simulink model "HDLRxPayload"  (R2024a)
settings: Solver=FixedStepDiscrete  StartTime=0.0  StopTime=stopTime  RelTol=1e-3
values from neighbouring files (symbols this model uses):
  payloadRxLLR = ofdmDemodulate(payloadTx, payloadBitsPerSubcarrier, payloadCyclicPrefixLen, nullIdx, payloadScramblerInit, true)    [testRxPayload.m]
  validIn = true(size(payloadRxLLR))    [testRxPayload.m]
undefined symbols (not defined in the file or in its folder): CONST, totalPayloadFecBlocks
libraries: hdlsllib x9, dspsrcs4 x8, HDL_ieee_8021513 x2, whdlutilities x1
settings Model: DataTypeOverride=Off  SimulationMode=accelerator  Creator=cotti  LastModifiedBy=cotti
settings OptimizationCC: BlockReduction=off  ConditionallyExecuteInputs=off  DefaultParameterBehavior=Inlined  InheritOutputTypeSmallerThanSingle=on
settings DebuggingCC: AlgebraicLoopMsg=error  ArtificialAlgebraicLoopMsg=error  SingleTaskRateTransMsg=error  UnconnectedInputMsg=warning  UnconnectedOutputMsg=warning  UnconnectedLineMsg=warning
settings HardwareCC: ProdBitPerPointer=32  ProdBitPerSizeT=32  ProdBitPerPtrDiffT=32  ProdLargestAtomicFloat=None  ProdIntDivRoundTo=Undefined  ProdEndianess=Unspecified  ProdWordSize=32  ProdHWDeviceType=ASIC/FPGA->ASIC/FPGA  TargetBitPerLong=64  TargetBitPerPointer=64  TargetBitPerSizeT=64  TargetBitPerPtrDiffT=64  TargetLongLongMode=on  TargetIntDivRoundTo=Zero  TargetEndianess=LittleEndian  TargetWordSize=64  TargetHWDeviceType=Custom Processor->MATLAB Host Computer  ProdEqTarget=off

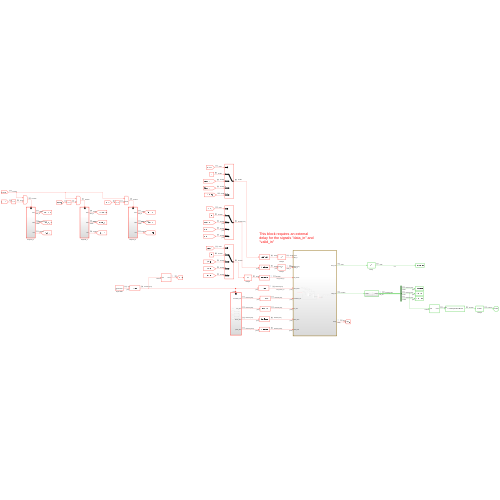
[thumbnail: Simulink's stored preview of the top-level diagram]
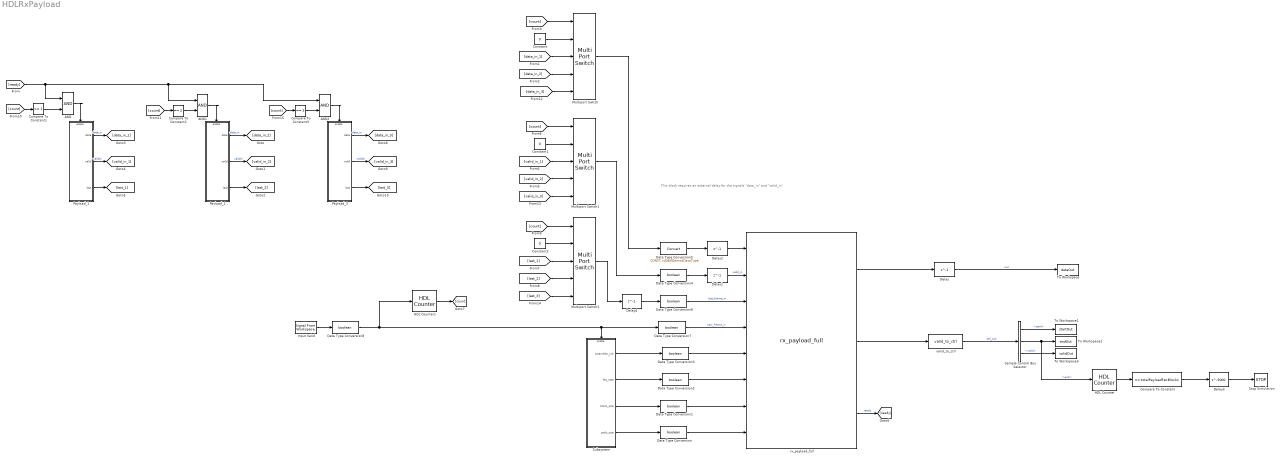
== system HDLRxPayload ==
  note: This block requires an external delay for the signals "data_in" and "valid_in"
  AND : Logic  IconShape=distinctive  AllPortsSameDT=off  OutDataTypeStr=boolean
  AND1 : Logic  IconShape=distinctive  AllPortsSameDT=off  OutDataTypeStr=boolean
  AND2 : Logic  IconShape=distinctive  AllPortsSameDT=off  OutDataTypeStr=boolean
  Compare To Constant : hdlsllib/Logic and Bit Operations/Compare To Constant  relop===  const=totalPayloadFecBlocks  OutDataTypeStr=boolean
  Compare To Constant1 : hdlsllib/Logic and Bit Operations/Compare To Constant  relop===  const=1  OutDataTypeStr=boolean
  Compare To Constant2 : hdlsllib/Logic and Bit Operations/Compare To Constant  relop===  const=2  OutDataTypeStr=boolean
  Compare To Constant3 : hdlsllib/Logic and Bit Operations/Compare To Constant  relop===  const=3  OutDataTypeStr=boolean
  Constant : Constant  Value=0  OutDataTypeStr=Inherit: Inherit via back propagation  SampleTime=-1
  Constant1 : Constant  Value=0  OutDataTypeStr=Inherit: Inherit via back propagation  SampleTime=-1
  Constant2 : Constant  Value=0  OutDataTypeStr=Inherit: Inherit via back propagation  SampleTime=-1
  Data Type Conversion{,1..4,6..8} (8 alike) : DataTypeConversion  OutDataTypeStr=boolean  SaturateOnIntegerOverflow=off  RndMeth=Floor
  Data Type Conversion5 : DataTypeConversion  OutDataTypeStr=CONST.rxQAMDemodDataType  SaturateOnIntegerOverflow=off  RndMeth=Floor
  Delay{,1..2,4} (4 alike) : Delay  DelayLength=1  InitialCondition=0  UseCircularBuffer=on
  Delay3 : Delay  DelayLength=5000  InitialCondition=0  UseCircularBuffer=on
  HDL Counter : hdlsllib/Sources/HDL Counter  CountType=Free running  CountInit=0  CountStep=1  CountMax=25  CountFromType=Initial value  CountFrom=0  CountResetPort=off  CountLoadPort=off  CountEnbPort=on  CountDirPort=off  CountHitOutputPort=off  CountDataType=Unsigned  CountWordLen=32  CountFracLen=0  CountSampTime=1
  HDL Counter1 : hdlsllib/Sources/HDL Counter  CountType=Free running  CountInit=0  CountStep=1  CountMax=25  CountFromType=Initial value  CountFrom=0  CountResetPort=off  CountLoadPort=off  CountEnbPort=on  CountDirPort=off  CountHitOutputPort=off  CountDataType=Unsigned  CountWordLen=8  CountFracLen=0  CountSampTime=1
  Input Valid : dspsrcs4/Signal From Workspace  X=newFrame  Ts=1/(2*CONST.fPHY)  nsamps=1  OutputAfterFinalValue=Setting to zero  ignoreOrWarnInputAndFrameLengths=off  OutputFrames=off
  Multiport Switch : MultiPortSwitch  DataPortOrder=Zero-based contiguous  Inputs=4  zeroidx=on  SaturateOnIntegerOverflow=off  InputSameDT=off
  Multiport Switch1 : MultiPortSwitch  DataPortOrder=Zero-based contiguous  Inputs=4  zeroidx=on  SaturateOnIntegerOverflow=off  InputSameDT=off
  Multiport Switch2 : MultiPortSwitch  DataPortOrder=Zero-based contiguous  Inputs=4  zeroidx=on  SaturateOnIntegerOverflow=off  InputSameDT=off
  Payload_1 : Subsystem  TreatAsAtomicUnit=on
  Payload_2 : Subsystem  TreatAsAtomicUnit=on
  Payload_3 : Subsystem  TreatAsAtomicUnit=on
  Sample Control Bus Selector : whdlutilities/Sample Control Bus Selector  OutputSignals=start,end,valid
  Stop Simulation : Stop
  Subsystem : Subsystem
  To Workspace : ToWorkspace  VariableName=dataOut  SampleTime=4/CONST.fPHY
      settings: Save2DSignal=2-D array (concatenate along first dimension)
  To Workspace1 : ToWorkspace  VariableName=startOut  SampleTime=4/CONST.fPHY
      settings: Save2DSignal=2-D array (concatenate along first dimension)
  To Workspace2 : ToWorkspace  VariableName=endOut  SampleTime=4/CONST.fPHY
      settings: Save2DSignal=2-D array (concatenate along first dimension)
  To Workspace3 : ToWorkspace  VariableName=validOut  SampleTime=4/CONST.fPHY
      settings: Save2DSignal=2-D array (concatenate along first dimension)
  rx_payload_full : HDL_ieee_8021513/rx_payload_full  SystemSampleTime=-1  VariantActivationTime=update diagram  AllowFlexibleInterface=on  Latency=0  AutoFrameSizeCalculation=off
      settings: SourceProductName=HDL IEEE 8021513
  valid_to_ctrl : HDL_ieee_8021513/valid_to_ctrl  SystemSampleTime=-1  VariantActivationTime=update diagram  AllowFlexibleInterface=on  Latency=0  AutoFrameSizeCalculation=off
      settings: SourceProductName=HDL IEEE 8021513
  wires:
  Sample Control Bus Selector/2 -> HDL Counter/1, To Workspace2/1  "<end>"
  Delay/1 -> To Workspace/1  "out"
  Sample Control Bus Selector/1 -> To Workspace1/1  "<start>"
  Sample Control Bus Selector/3 -> To Workspace3/1  "<valid>"
  valid_to_ctrl/1 -> Sample Control Bus Selector/1  "ctrl_out"
  rx_payload_full/2 -> valid_to_ctrl/1
  rx_payload_full/1 -> Delay/1
  Data Type Conversion/1 -> rx_payload_full/8
  Data Type Conversion1/1 -> rx_payload_full/7
  Data Type Conversion2/1 -> rx_payload_full/6
  Data Type Conversion3/1 -> rx_payload_full/5
  Data Type Conversion4/1 -> Delay1/1
  Data Type Conversion5/1 -> Delay2/1
  Data Type Conversion6/1 -> rx_payload_full/3  "last_frame_in"
  Data Type Conversion7/1 -> rx_payload_full/4  "new_frame_in"
  Delay2/1 -> rx_payload_full/1
  Delay1/1 -> rx_payload_full/2  "valid_in"
  HDL Counter/1 -> Compare To Constant/1
  Compare To Constant/1 -> Delay3/1
  Subsystem/1(scrambler_init) -> Data Type Conversion3/1
  Subsystem/2(fec_rate) -> Data Type Conversion2/1
  Subsystem/3(block_size) -> Data Type Conversion1/1
  Subsystem/4(psdu_size) -> Data Type Conversion/1
  Input Valid/1 -> Data Type Conversion8/1
  Delay3/1 -> Stop Simulation/1
  Payload_2/1(data) -> [data_in_2]  "data_in"
  Payload_2/2(valid) -> [valid_in_2]  "validIn"
  Payload_2/3(last) -> [last_2]
  Payload_1/1(data) -> [data_in_1]  "data_in"
  Payload_1/2(valid) -> [valid_in_1]  "validIn"
  Payload_1/3(last) -> [last_1]
  rx_payload_full/3 -> [ready]  "ready"
  [data_in_1] -> Multiport Switch/3
  [data_in_2] -> Multiport Switch/4
  Constant/1 -> Multiport Switch/2
  Multiport Switch/1 -> Data Type Conversion5/1
  HDL Counter1/1 -> [count]
  [count] -> Multiport Switch/1
  Constant1/1 -> Multiport Switch1/2
  [valid_in_2] -> Multiport Switch1/4
  [valid_in_1] -> Multiport Switch1/3
  [count] -> Multiport Switch1/1
  Constant2/1 -> Multiport Switch2/2
  [last_2] -> Multiport Switch2/4
  [last_1] -> Multiport Switch2/3
  [count] -> Multiport Switch2/1
  Multiport Switch2/1 -> Delay4/1
  Multiport Switch1/1 -> Data Type Conversion4/1
  AND/1 -> Payload_1/Enable
  AND1/1 -> Payload_2/Enable
  Compare To Constant1/1 -> AND/2
  Compare To Constant2/1 -> AND1/2
  [count] -> Compare To Constant1/1
  [count] -> Compare To Constant2/1
  Data Type Conversion8/1 -> HDL Counter1/1, Subsystem/Enable, Data Type Conversion7/1
  [data_in_3] -> Multiport Switch/5
  [valid_in_3] -> Multiport Switch1/5
  [last_3] -> Multiport Switch2/5
  Payload_3/3(last) -> [last_3]
  Payload_3/1(data) -> [data_in_3]  "data_in"
  Payload_3/2(valid) -> [valid_in_3]  "validIn"
  Compare To Constant3/1 -> AND2/2
  [count] -> Compare To Constant3/1
  [ready] -> AND/1, AND2/1, AND1/1
  AND2/1 -> Payload_3/Enable
  Delay4/1 -> Data Type Conversion6/1

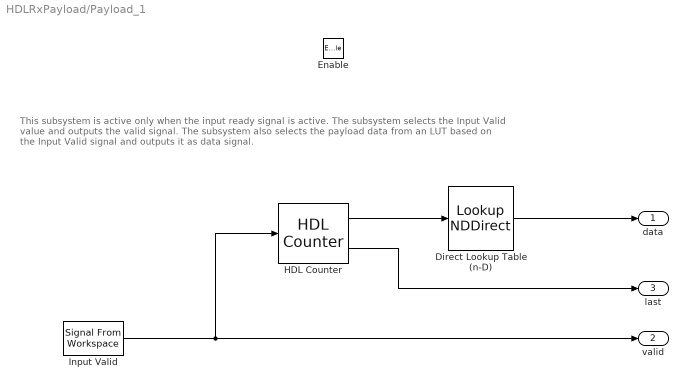
== system HDLRxPayload/Payload_1 ==
  note: This subsystem is active only when the input ready signal is active. The subsystem selects the Input Valid value and outputs the valid signal.
      | The subsystem also selects the payload data from an LUT based on the Input Valid signal and outputs it as data signal.
  Enable : EnablePort
  Direct Lookup Table (n-D) : LookupNDDirect  NumberOfTableDimensions=1  Table=payloadRxLLR{1}  DiagnosticForOutOfRangeInput=Error  TableDataTypeStr=double
  HDL Counter : hdlsllib/Sources/HDL Counter  CountType=Count limited  CountInit=0  CountStep=1  CountMax=length(payloadRxLLR{1}) -1  CountFromType=Initial value  CountFrom=0  CountResetPort=off  CountLoadPort=off  CountEnbPort=on  CountDirPort=off  CountHitOutputPort=on  CountDataType=Unsigned  CountWordLen=nextpow2(length(payloadRxLLR{1}))  CountFracLen=0  CountSampTime=1
  Input Valid : dspsrcs4/Signal From Workspace  X=validIn{1}  Ts=1/(2*CONST.fPHY)  nsamps=1  OutputAfterFinalValue=Setting to zero  ignoreOrWarnInputAndFrameLengths=off  OutputFrames=off
  data : Outport  InitialOutput=0  VectorParamsAs1DForOutWhenUnconnected=off
  valid : Outport  Port=2  InitialOutput=0  VectorParamsAs1DForOutWhenUnconnected=off
  last : Outport  Port=3  VectorParamsAs1DForOutWhenUnconnected=off
  wires:
  HDL Counter/1 -> Direct Lookup Table (n-D)/1
  Direct Lookup Table (n-D)/1 -> data/1
  Input Valid/1 -> valid/1, HDL Counter/1
  HDL Counter/2 -> last/1

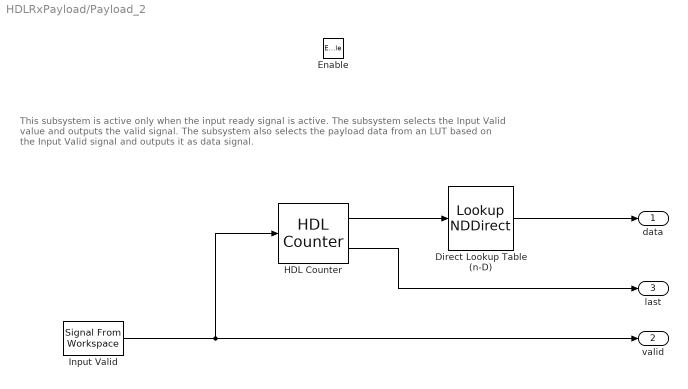
== system HDLRxPayload/Payload_2 ==
  note: This subsystem is active only when the input ready signal is active. The subsystem selects the Input Valid value and outputs the valid signal.
      | The subsystem also selects the payload data from an LUT based on the Input Valid signal and outputs it as data signal.
  Enable : EnablePort
  Direct Lookup Table (n-D) : LookupNDDirect  NumberOfTableDimensions=1  Table=payloadRxLLR{2}  DiagnosticForOutOfRangeInput=Error  TableDataTypeStr=double
  HDL Counter : hdlsllib/Sources/HDL Counter  CountType=Count limited  CountInit=0  CountStep=1  CountMax=length(payloadRxLLR{2}) -1  CountFromType=Initial value  CountFrom=0  CountResetPort=off  CountLoadPort=off  CountEnbPort=on  CountDirPort=off  CountHitOutputPort=on  CountDataType=Unsigned  CountWordLen=nextpow2(length(payloadRxLLR{2}))  CountFracLen=0  CountSampTime=1
  Input Valid : dspsrcs4/Signal From Workspace  X=validIn{2}  Ts=1/(2*CONST.fPHY)  nsamps=1  OutputAfterFinalValue=Setting to zero  ignoreOrWarnInputAndFrameLengths=off  OutputFrames=off
  data : Outport  InitialOutput=0  VectorParamsAs1DForOutWhenUnconnected=off
  valid : Outport  Port=2  InitialOutput=0  VectorParamsAs1DForOutWhenUnconnected=off
  last : Outport  Port=3  VectorParamsAs1DForOutWhenUnconnected=off
  wires:
  HDL Counter/1 -> Direct Lookup Table (n-D)/1
  Direct Lookup Table (n-D)/1 -> data/1
  Input Valid/1 -> valid/1, HDL Counter/1
  HDL Counter/2 -> last/1

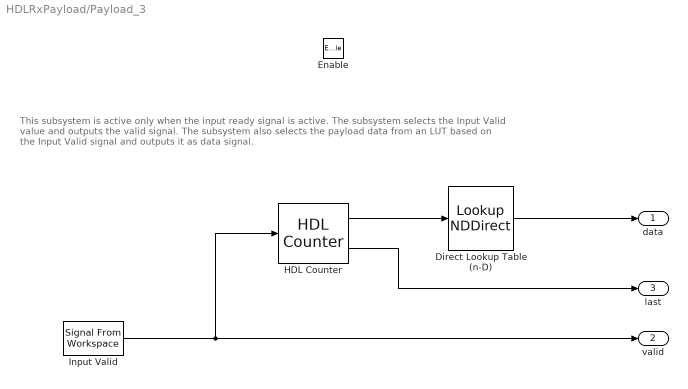
== system HDLRxPayload/Payload_3 ==
  note: This subsystem is active only when the input ready signal is active. The subsystem selects the Input Valid value and outputs the valid signal.
      | The subsystem also selects the payload data from an LUT based on the Input Valid signal and outputs it as data signal.
  Enable : EnablePort
  Direct Lookup Table (n-D) : LookupNDDirect  NumberOfTableDimensions=1  Table=payloadRxLLR{3}  DiagnosticForOutOfRangeInput=Error  TableDataTypeStr=double
  HDL Counter : hdlsllib/Sources/HDL Counter  CountType=Count limited  CountInit=0  CountStep=1  CountMax=length(payloadRxLLR{3}) -1  CountFromType=Initial value  CountFrom=0  CountResetPort=off  CountLoadPort=off  CountEnbPort=on  CountDirPort=off  CountHitOutputPort=on  CountDataType=Unsigned  CountWordLen=nextpow2(length(payloadRxLLR{3}))  CountFracLen=0  CountSampTime=1
  Input Valid : dspsrcs4/Signal From Workspace  X=validIn{3}  Ts=1/(2*CONST.fPHY)  nsamps=1  OutputAfterFinalValue=Setting to zero  ignoreOrWarnInputAndFrameLengths=off  OutputFrames=off
  data : Outport  InitialOutput=0  VectorParamsAs1DForOutWhenUnconnected=off
  valid : Outport  Port=2  InitialOutput=0  VectorParamsAs1DForOutWhenUnconnected=off
  last : Outport  Port=3  VectorParamsAs1DForOutWhenUnconnected=off
  wires:
  HDL Counter/1 -> Direct Lookup Table (n-D)/1
  Direct Lookup Table (n-D)/1 -> data/1
  Input Valid/1 -> valid/1, HDL Counter/1
  HDL Counter/2 -> last/1

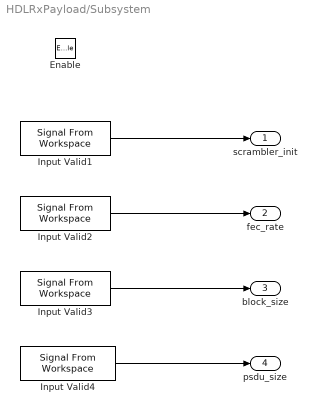
== system HDLRxPayload/Subsystem ==
  Enable : EnablePort
  Input Valid1 : dspsrcs4/Signal From Workspace  X=scramblerInitLSB  Ts=1/(2*CONST.fPHY)  nsamps=1  OutputAfterFinalValue=Setting to zero  ignoreOrWarnInputAndFrameLengths=off  OutputFrames=off
  Input Valid2 : dspsrcs4/Signal From Workspace  X=fecRateLSB  Ts=1/(2*CONST.fPHY)  nsamps=1  OutputAfterFinalValue=Setting to zero  ignoreOrWarnInputAndFrameLengths=off  OutputFrames=off
  Input Valid3 : dspsrcs4/Signal From Workspace  X=blockSizeLSB  Ts=1/(2*CONST.fPHY)  nsamps=1  OutputAfterFinalValue=Setting to zero  ignoreOrWarnInputAndFrameLengths=off  OutputFrames=off
  Input Valid4 : dspsrcs4/Signal From Workspace  X=psduSizeLSB  Ts=1/(2*CONST.fPHY)  nsamps=1  OutputAfterFinalValue=Setting to zero  ignoreOrWarnInputAndFrameLengths=off  OutputFrames=off
  scrambler_init : Outport
  fec_rate : Outport  Port=2
  block_size : Outport  Port=3
  psdu_size : Outport  Port=4
  wires:
  Input Valid3/1 -> block_size/1
  Input Valid1/1 -> scrambler_init/1
  Input Valid4/1 -> psdu_size/1
  Input Valid2/1 -> fec_rate/1
